simulink model "question2222"  (R2023a)
settings: Solver=VariableStepAuto  StartTime=0.0  StopTime=5  RelTol=1e-3
values from neighbouring files (symbols this model uses):
  A = [0 1 0;0 0 1;0 0 0]    [test.m]
  B = [0 ;0;1 ]    [test.m]
  C = [1 0 0 0 ... (first row only)    [test.m]
  K = place(A,B,polesoute)    [test.m]
  L = L'    [test.m]
settings Model: Creator=haoyuan  LastModifiedBy=haoyuan

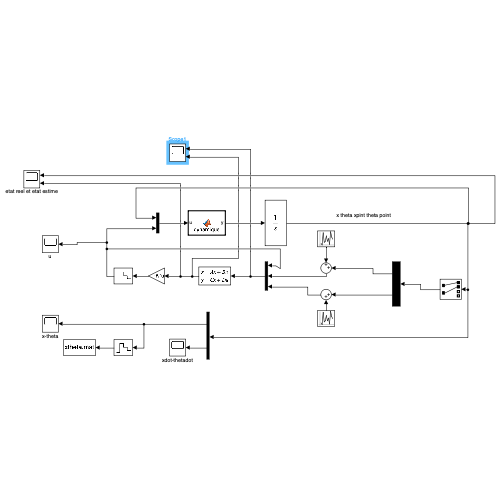
[thumbnail: Simulink's stored preview of the top-level diagram]
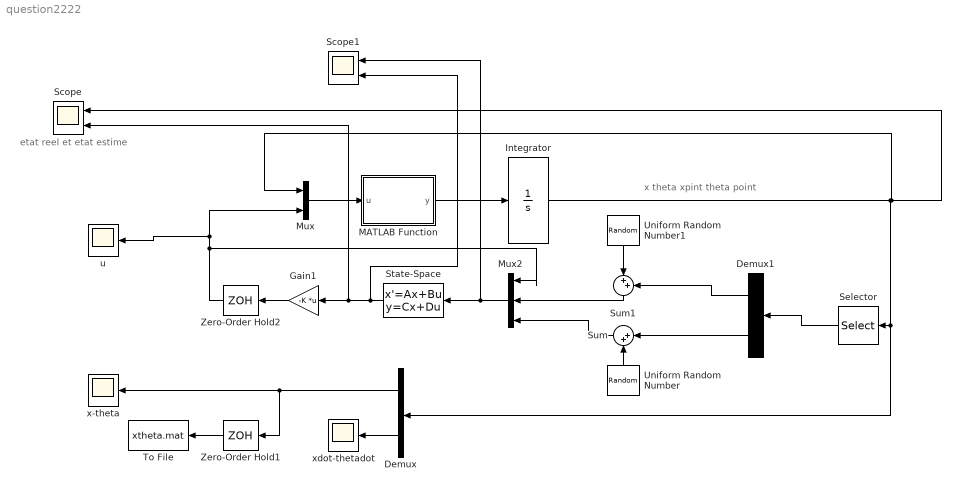
== system question2222 ==
  note: etat reel et etat estime
  note: x theta xpint theta point
  Demux : Demux  Outputs=2
  Demux1 : Demux  Outputs=2
  Gain1 : Gain  Gain=-K  Multiplication=Matrix(K*u)
  Integrator : Integrator  InitialCondition=[0;0.3;0;0]
  MATLAB Function : MATLAB Function  TreatAsAtomicUnit=on
  Mux : Mux  Inputs=2
  Mux2 : Mux  Inputs=3
  Scope : Scope  NumInputPorts=2
  Scope1 : Scope  NumInputPorts=2
  Selector : Selector  InputPortWidth=4  IndexOptions=Index vector (dialog)  Indices=[1 2]  OutputSizes=1
  State-Space : StateSpace  A=A-L*C  B=[B L]  C=eye(4)  D=[0 0 0 0;0 0 0 0;0 0 0 0;0 0 0]  InitialCondition=0
  Sum : Sum  Inputs=|++
  Sum1 : Sum  Inputs=|++
  To File : ToFile  Filename=xtheta.mat  SaveFormat=Timeseries  SampleTime=0.01
  Uniform Random Number : UniformRandomNumber  Minimum=-0.02  Maximum=0.02  SampleTime=1/1000
  Uniform Random Number1 : UniformRandomNumber  Minimum=-0.02  Maximum=0.02  SampleTime=1/100
  Zero-Order Hold1 : ZeroOrderHold  SampleTime=0.01
  Zero-Order Hold2 : ZeroOrderHold  SampleTime=0.01
  u : Scope
  x-theta : Scope
  xdot-thetadot : Scope
  wires:
  Demux/1 -> Zero-Order Hold1/1, x-theta/1
  Zero-Order Hold1/1 -> To File/1
  Demux/2 -> xdot-thetadot/1
  Mux/1 -> MATLAB Function/1(u)
  MATLAB Function/1(y) -> Integrator/1
  Mux2/1 -> Scope1/1, State-Space/1
  Integrator/1 -> Scope/1, Mux/1, Demux/1, Selector/1
  Zero-Order Hold2/1 -> u/1, Mux/2, Mux2/1
  Gain1/1 -> Zero-Order Hold2/1
  State-Space/1 -> Scope1/2, Scope/2, Gain1/1
  Selector/1 -> Demux1/1
  Demux1/2 -> Sum/1
  Uniform Random Number/1 -> Sum/2
  Sum1/1 -> Mux2/2
  Sum/1 -> Mux2/3
  Uniform Random Number1/1 -> Sum1/1
  Demux1/1 -> Sum1/2

== matlab function question2222/MATLAB Function ==
  data: u input; y output
function y = dynamique(u)
% fonction définissant la dynamique du système: renvoie f(X,U) avec X
% l'état, et U la variable de commande physique (composante T de la force
% appliquée au chariot)

x= u(1); %position du chariot
theta= u(2); %inclinaison de la barre
xdot= u(3); % vitesse du chariot
thetadot= u(4); % vitesse angulaire de la barre
T= u(5); % force appliquée au chariot

% Defintion des paramètres du système
m= 0.2; % masse de la barre
M= 1; % masse totale (chariot + barre)
l= 0.2 % demi-longueur de la barre
J=  m*l^2/3; % inertie de la barre
g= 9.81; % cste de gravité
mu= 0.005; % coeff. de frottement visqueux barre
tau= 0.2; % coeff. de frottement visqueux chariot

% Calcul des dérivées secondes
Delta_theta= M*(J+m*l^2)-m^2*l^2*(cos(theta))^2;
disp(Delta_theta);
%2*2 2*1
xthetaddot=1/Delta_theta*[J+m*l^2 -m*l*cos(theta);-m*l*cos(theta) M]*...
    [T+m*l*thetadot^2*sin(theta)-tau*xdot;m*g*l*sin(theta)-mu*thetadot];
%Calcul de f
y = [xdot;thetadot;xthetaddot];
